simulink model "Task3_MaximumPowerPointTracking"  (R2026a)
settings: Solver=VariableStepAuto  StopTime=100
values from neighbouring files (symbols this model uses):
  Ts = 0.1    [profileData.mat]
libraries: fl_lib x6, nesl_utility x6, simulink x4, ee_lib x2
settings Model: Creator=gdudgeon  LastModifiedBy=gracew
settings SimscapeCC: SimscapeNominalValues="[{\"value\":\"1\",\"unit\":\"A\"},{\"value\":\"1\",\"unit\":\"bar\"},{\"value\":\"1\",\"unit\":\"cm^2\"},{\"value\":\"1\",\"unit\":\"cm^3/s\"},{\"value\":\"1\",\"unit\":\"kJ/kg\"},{\"value\":\"1\",\"unit\":\"kW\"},{\"value\":\"1\",\"unit\":\"l\"},{\"value\":\"1\",\"unit\":\"N\"},{\"value\":\"1\",\"unit\":\"N*m\"},{\"value\":\"1\",\"unit\":\"V\"}]"  SimscapeLogType=none  SimscapeLogDataHistory=5000.0

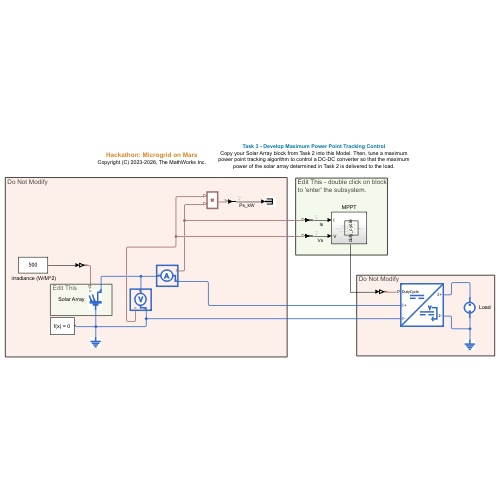
[thumbnail: Simulink's stored preview of the top-level diagram]
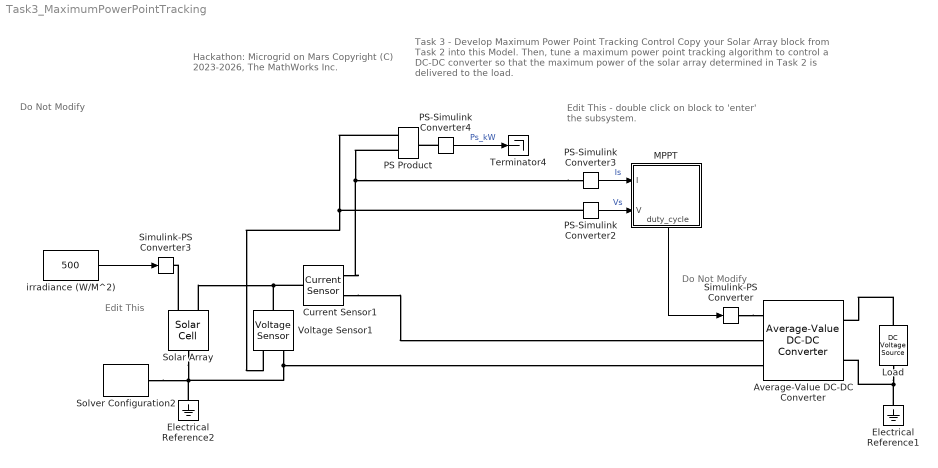
== system Task3_MaximumPowerPointTracking ==
  note: Edit This
  note: Do Not Modify
  note: Edit This - double click on block
      | to 'enter' the subsystem.
  note: Do Not Modify
  note: Task 3 - Develop Maximum Power Point Tracking Control
      | Copy your Solar Array block from Task 2 into this Model. Then, tune a maximum power point tracking algorithm to control a DC-DC converter so that the maximum power of the solar array determined in Task 2 is delivered to the load.
  note: Hackathon: Microgrid on Mars
      | Copyright (C) 2023-2026, The MathWorks Inc.
  " irradiance (W/M^2)" : Constant  Value=500
  Average-Value DC-DC Converter : ee_lib/Semiconductors & Converters/Converters/Average-Value DC-DC Converter  implementation_option=ee.enum.converters.implementation.behavioral  converter_type=ee.enum.converters.dcdctype.buckboost  control_option=ee.enum.converters.controlinput.dutycycle  efficiency_option=ee.enum.converters.efficiency.constant  efficiency_fixed=100  i_vec=[0, 2, 5] A  efficiency_vec=[90, 95, 98]  Lf=1e-6 H  Rl=0 Ohm  Cf=1e-7 F  Rc=1e-6 Ohm  iL_specify=off  iL_priority=High  iL=0 A  iL_nominal_specify=off  iL_nominal_value=1  iL_nominal_unit=A  vc_specify=off  vc_priority=High  vc=0 V  vc_nominal_specify=off  vc_nominal_value=1  vc_nominal_unit=V
  Current Sensor1 : fl_lib/Electrical/Electrical Sensors/Current Sensor
  Electrical Reference1 : fl_lib/Electrical/Electrical Elements/Electrical Reference
  Electrical Reference2 : fl_lib/Electrical/Electrical Elements/Electrical Reference
  Load : fl_lib/Electrical/Electrical Sources/DC Voltage Source  v0=500 V
  MPPT : Subsystem
      settings: PortSchema="{\"entries\":[{\"content\":{\"sides\":[{\"content\":{\"connectorIds\":[\"In1\",\"In2\"]},\"type\":\"ConnectorPlacement.EquallySpacedRectSide\",\"uuid\":\"38bd0aeb-e74d-4899-bfbb-86ccd5f95d4f\"},{\"content\":{\"side\":\"RIGHT\"},\"type\":\"ConnectorPlacement.EquallySpacedRectSide\",\"uuid\":\"60d4d859-7951-4137-a4d3-aa9c7dbc0cca\"},{\"content\":{\"side\":\"TOP\"},\"type\":\"ConnectorPlacement.EquallySpacedRectSide\",\"uuid\":\"2b4b2d3e-d6d6-4128-a276-e12099a85009\"},{\"content\":{\"connectorIds\":[\"Out1\"],\"side\":\"BOTTOM\"},\"type\":\"ConnectorPlacement.EquallySpacedRectSide\",\"uuid\":\"409b20ff-1438-4235-89e6-0fc7ac87e62f\"}]},\"type\":\"ConnectorPlacement.EquallySpacedConnector\",\"uuid\":\"dc5f0d06-624a-4535-b1c9-b0abe4535c5f\"}],\"packageUris\":[\"http://schema.mathworks.com/mf0/Connector/R2020b\"],\"version\":\"1.0\"}"
  PS Product : fl_lib/Physical Signals/Functions/PS Product
  PS-Simulink Converter2 : nesl_utility/PS-Simulink Converter  PhysicalDomain=network_engine_domain  SubClassName=ps_output  LeftPortType=input  RightPortType=output  PseudoPeriodic=off  Frequencies=[]  VectorFormat=inherit  Unit=inherit  AffineConversion=off
  PS-Simulink Converter3 : nesl_utility/PS-Simulink Converter  PhysicalDomain=network_engine_domain  SubClassName=ps_output  LeftPortType=input  RightPortType=output  PseudoPeriodic=off  Frequencies=[]  VectorFormat=inherit  Unit=inherit  AffineConversion=off
  PS-Simulink Converter4 : nesl_utility/PS-Simulink Converter  PhysicalDomain=network_engine_domain  SubClassName=ps_output  LeftPortType=input  RightPortType=output  PseudoPeriodic=off  Frequencies=[]  VectorFormat=inherit  Unit=kW  AffineConversion=off
  Simulink-PS Converter : nesl_utility/Simulink-PS Converter  PhysicalDomain=network_engine_domain  SubClassName=ps_input  LeftPortType=input  RightPortType=output  PseudoPeriodic=off  Frequencies=[]  NoiseDistribution=none  NoiseParameters=[]  Unit=1  AffineConversion=off  FilteringAndDerivatives=provide  SimscapeFilterOrder=1  InputFilterTimeConstant=0.001  UdotUserProvided=0
  Simulink-PS Converter3 : nesl_utility/Simulink-PS Converter  PhysicalDomain=network_engine_domain  SubClassName=ps_input  LeftPortType=input  RightPortType=output  PseudoPeriodic=off  Frequencies=[]  NoiseDistribution=none  NoiseParameters=[]  Unit=W/m^2  AffineConversion=off  FilteringAndDerivatives=provide  SimscapeFilterOrder=1  InputFilterTimeConstant=0.001  UdotUserProvided=0
  Solar Array : ee_lib/Sources/Solar Cell  prm=1  Isc=10.6 A  Voc=0.61 V  Is=1e-6 A  Is2=0 A  Iph=7.34 A  Ir0=500 W/m^2  ec=1.5  N2=2  Rs=0 Ohm  Rp=inf Ohm  N_series=1000  N_parallel=10  TIPH1=0 1/K  EG=1.11 eV  TXIS1=3  TXIS2=3  TRS1=0  TRP1=0  Tmeas=25 degC  TFIXED=25 degC  thermal_mass=100 J/K  initial_temperature=25 degC
  Solver Configuration2 : nesl_utility/Solver Configuration  PhysicalDomain=network_engine_domain  SubClassName=solver  LeftPortType=input  RightPortType=generic  Tones=[]  Harmonics=[]  SimulateNoise=off  Profile=off  UseLocalSampling=off  EnableSwitchedLinearOptims=on  FrequencyDomain=off  UseCCode=off  RelTol=0.001  AbsTol=0.001  MinStep=1e-09  ToWorkspace=off  RevertToSquareIcSolve=off  NumHomotopyIterations=100  PhasorMode=off  PhasorModeNumHarmonics=1  ConsistencySolver=NEWTON_XTOL_AFTER_FTOL  CanonicalOrdering=UNORDERED  OptimizeIntermediates=UNOPTIMIZED  IndexReductionMethod=None  DoDC=off  ResidualTolerance=1e-09  ConsistencyTolSource=GLOBAL  ConsistencyAbsTol=0.001  ConsistencyRelTol=0.001  ConsistencyTolFactor=0.001  UseLocalSolver=on  LocalSolverChoice=NE_BACKWARD_EULER_ADVANCER  ResolveIndetEquations=off  FunctionEvalNumThread=1  LocalSolverSampleTime=Ts  DoFixedCost=on  MaxNonlinIter=1  MaxModeIter=2  ComputeImpulses=off  ImpulseIterations=2  LinearAlgebra=Sparse  LinearAlgebraNumThread=0  EquationFormulation=NE_TIME_EF  DelaysMemoryBudget=1024  AutomaticFiltering=off  FilteringTimeConstant=0.001  PartitionStorageMethod=AS_NEEDED  PartitionMemoryBudget=1024  PartitionMethod=ROBUST  MultibodyUseLocalSolver=off  MultibodyLocalSolverChoice=ODE1  MultibodyLocalSolverSampleTime=0.001
  Terminator4 : Terminator
  Voltage Sensor1 : fl_lib/Electrical/Electrical Sensors/Voltage Sensor
  wires:
  MPPT/1(duty_cycle) -> Simulink-PS Converter/1
  " irradiance (W/M^2)"/1 -> Simulink-PS Converter3/1
  PS-Simulink Converter2/1 -> MPPT/2(V)  "Vs"
  PS-Simulink Converter3/1 -> MPPT/1(I)  "Is"
  PS-Simulink Converter4/1 -> Terminator4/1  "Ps_kW"
  connections:
  Current Sensor1/LConn1 -- Solar Array/LConn2 -- Voltage Sensor1/LConn1
  Average-Value DC-DC Converter/RConn2 -- Load/RConn1 -- Electrical Reference1/LConn1
  PS-Simulink Converter2/LConn1 -- Voltage Sensor1/RConn1 -- PS Product/LConn1
  Solver Configuration2/RConn1 -- Voltage Sensor1/RConn2 -- Average-Value DC-DC Converter/LConn3 -- Solar Array/RConn1 -- Electrical Reference2/LConn1
  PS-Simulink Converter3/LConn1 -- Current Sensor1/RConn1 -- PS Product/LConn2
  PS-Simulink Converter4/LConn1 -- PS Product/RConn1
  Simulink-PS Converter/RConn1 -- Average-Value DC-DC Converter/LConn1
  Current Sensor1/RConn2 -- Average-Value DC-DC Converter/LConn2
  Load/LConn1 -- Average-Value DC-DC Converter/RConn1
  Solar Array/LConn1 -- Simulink-PS Converter3/RConn1

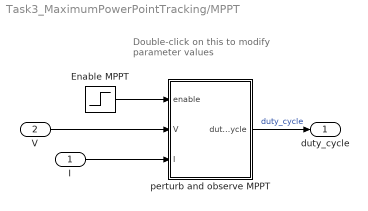
== system Task3_MaximumPowerPointTracking/MPPT ==
  note: Double-click on this
      | to modify parameter values
  I : Inport
  V : Inport  Port=2
  Enable MPPT : Step  Time=0.1  SampleTime=0
  perturb and observe MPPT : Subsystem  mask{Dinit=0.7, Dmax=0.7, Dmin=0.7, DeltaD=1}
      mask prompts: Dinit "Initial value for D output (Dinit)"; Dmax "Upper limit for D (Dmax)"; Dmin "Lower limit for D (Dmin)"; DeltaD "Increment value used to increase/decrease (DeltaD)"
  duty_cycle : Outport
  wires:
  V/1 -> perturb and observe MPPT/2(V)
  Enable MPPT/1 -> perturb and observe MPPT/1(enable)
  I/1 -> perturb and observe MPPT/3(I)
  perturb and observe MPPT/1(duty_cycle) -> duty_cycle/1  "duty_cycle"

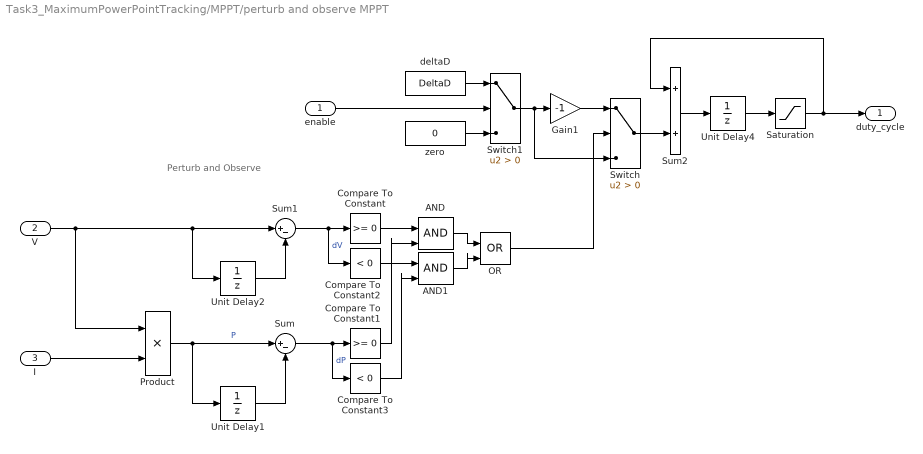
== system Task3_MaximumPowerPointTracking/MPPT/perturb and observe MPPT ==
  note: Perturb and Observe
  enable : Inport
  V : Inport  Port=2
  I : Inport  Port=3
  AND : Logic  IconShape=distinctive  AllPortsSameDT=off  OutDataTypeStr=boolean
  AND1 : Logic  IconShape=distinctive  AllPortsSameDT=off  OutDataTypeStr=boolean
  Compare To Constant : simulink/Logic and Bit Operations/Compare To Constant  relop=>=  const=0  OutDataTypeStr=boolean
  Compare To Constant1 : simulink/Logic and Bit Operations/Compare To Constant  relop=>=  const=0  OutDataTypeStr=boolean
  Compare To Constant2 : simulink/Logic and Bit Operations/Compare To Constant  relop=<  const=0  OutDataTypeStr=boolean
  Compare To Constant3 : simulink/Logic and Bit Operations/Compare To Constant  relop=<  const=0  OutDataTypeStr=boolean
  Gain1 : Gain  Gain=-1
  OR : Logic  Operator=OR  IconShape=distinctive  AllPortsSameDT=off  OutDataTypeStr=boolean
  Product : Product
  Saturation : Saturate  UpperLimit=Dmax  LowerLimit=Dmin
  Sum : Sum  Inputs=|+-
  Sum1 : Sum  Inputs=|+-
  Sum2 : Sum
  Switch : Switch  Criteria=u2 > Threshold  SaturateOnIntegerOverflow=off  InputSameDT=off
  Switch1 : Switch  Criteria=u2 > Threshold  SaturateOnIntegerOverflow=off  InputSameDT=off
  Unit Delay1 : UnitDelay  SampleTime=-1
  Unit Delay2 : UnitDelay  SampleTime=-1
  Unit Delay4 : UnitDelay  InitialCondition=Dinit  SampleTime=Ts
  deltaD : Constant  Value=DeltaD
  zero : Constant  Value=0
  duty_cycle : Outport
  wires:
  Unit Delay1/1 -> Sum/2
  V/1 -> Product/1, Unit Delay2/1, Sum1/1
  Switch/1 -> Sum2/2
  Compare To Constant/1 -> AND/1
  Switch1/1 -> Switch/3, Gain1/1
  AND/1 -> OR/1
  OR/1 -> Switch/2
  Gain1/1 -> Switch/1
  Sum/1 -> Compare To Constant3/1, Compare To Constant1/1  "dP"
  deltaD/1 -> Switch1/1
  Saturation/1 -> duty_cycle/1, Sum2/1
  Compare To Constant1/1 -> AND/2
  Sum1/1 -> Compare To Constant2/1, Compare To Constant/1  "dV"
  Compare To Constant2/1 -> AND1/1
  Product/1 -> Unit Delay1/1, Sum/1  "P"
  Compare To Constant3/1 -> AND1/2
  I/1 -> Product/2
  enable/1 -> Switch1/2
  Unit Delay2/1 -> Sum1/2
  AND1/1 -> OR/2
  zero/1 -> Switch1/3
  Sum2/1 -> Unit Delay4/1
  Unit Delay4/1 -> Saturation/1
